simulink model "Report_13_state_feedback_observer"  (R2022a)
settings: Solver=FixedStepAuto  StartTime=0.0  StopTime=10.0  FixedStep=1e-3  RelTol=1e-3
settings Model: Creator=takahiro  LastModifiedBy=takahiro

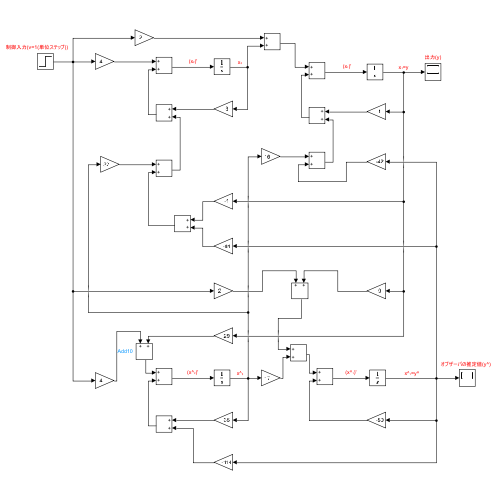
[thumbnail: Simulink's stored preview of the top-level diagram]
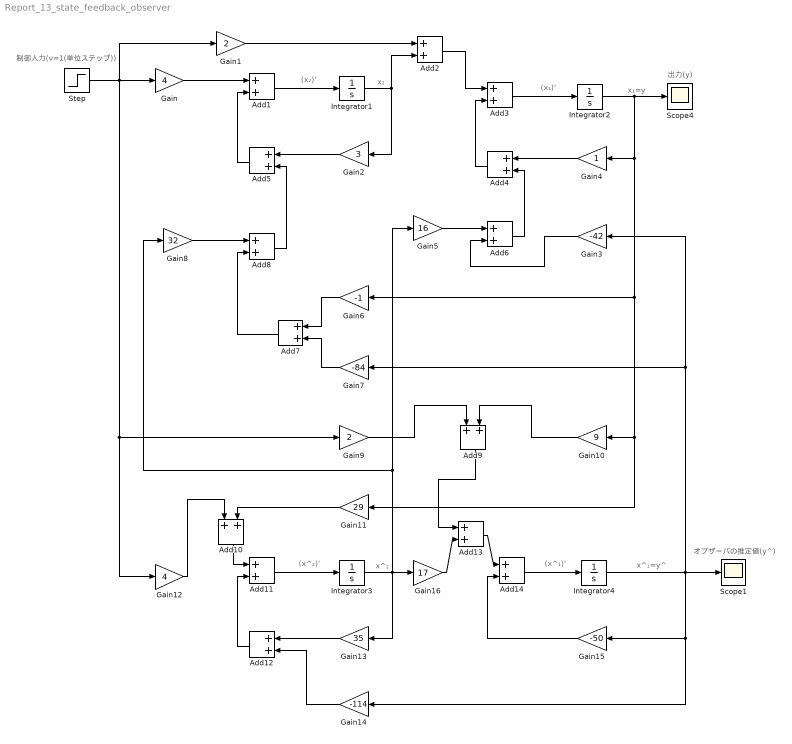
== system Report_13_state_feedback_observer ==
  note: 制御入力(v=1(単位ステップ))
  note: 出力(y)
  note: x₁=y
  note: (x₁)'
  note: x₂
  note: (x₂)'
  note: x^₁=y^
  note: (x^₁)'
  note: x^₂
  note: (x^₂)'
  note: オブザーバの推定値(y^)
  Add{1..14} (14 alike) : Sum
  Gain : Gain  Gain=4
  Gain1 : Gain  Gain=2
  Gain10 : Gain  Gain=9
  Gain11 : Gain  Gain=29
  Gain12 : Gain  Gain=4
  Gain13 : Gain  Gain=35
  Gain14 : Gain  Gain=-114
  Gain15 : Gain  Gain=-50
  Gain16 : Gain  Gain=17
  Gain2 : Gain  Gain=3
  Gain3 : Gain  Gain=-42
  Gain4 : Gain
  Gain5 : Gain  Gain=16
  Gain6 : Gain  Gain=-1
  Gain7 : Gain  Gain=-84
  Gain8 : Gain  Gain=32
  Gain9 : Gain  Gain=2
  Integrator{1..4} (4 alike) : Integrator
  Scope1 : Scope
  Scope4 : Scope
  Step : Step  Time=10  Before=1  SampleTime=0
  wires:
  Step/1 -> Gain12/1, Gain9/1, Gain1/1, Gain/1
  Gain/1 -> Add1/1
  Add1/1 -> Integrator1/1
  Integrator1/1 -> Gain2/1, Add2/2
  Gain1/1 -> Add2/1
  Add2/1 -> Add3/1
  Add3/1 -> Integrator2/1
  Integrator2/1 -> Gain6/1, Gain11/1, Gain10/1, Gain4/1, Scope4/1
  Gain4/1 -> Add4/1
  Add4/1 -> Add3/2
  Gain2/1 -> Add5/1
  Add5/1 -> Add1/2
  Gain3/1 -> Add6/2
  Add6/1 -> Add4/2
  Gain5/1 -> Add6/1
  Gain6/1 -> Add7/1
  Gain7/1 -> Add7/2
  Add7/1 -> Add8/2
  Add8/1 -> Add5/2
  Gain8/1 -> Add8/1
  Gain9/1 -> Add9/1
  Gain10/1 -> Add9/2
  Gain11/1 -> Add10/2
  Gain12/1 -> Add10/1
  Add10/1 -> Add11/1
  Add11/1 -> Integrator3/1
  Gain13/1 -> Add12/1
  Gain14/1 -> Add12/2
  Add12/1 -> Add11/2
  Add9/1 -> Add13/1
  Integrator3/1 -> Gain8/1, Gain5/1, Gain16/1, Gain13/1
  Add13/1 -> Add14/1
  Add14/1 -> Integrator4/1
  Gain15/1 -> Add14/2
  Integrator4/1 -> Gain7/1, Gain3/1, Gain14/1, Gain15/1, Scope1/1
  Gain16/1 -> Add13/2
